simulink model "accumulator"  (R2023b)
settings: Solver=FixedStepAuto  StartTime=0.0  StopTime=10.0  RelTol=1e-3
libraries: c280xlib x26, c2837xDlib x13, canmsglib x8
settings Model: ExtModeTrigDuration=8  Creator=steve  LastModifiedBy=lukeh
settings OptimizationCC: DefaultUnderspecifiedDataType=single  EnhancedBackFolding=on  PassReuseOutputArgsAs=Individual arguments  MaxStackSize=1024  OptimizeBlockOrder=speed  DifferentSizesBufferReuse=on  OptimizationCustomize=off  DenormalBehavior=FlushToZero  EfficientTunableParamExpr=on
settings DebuggingCC: ParameterTunabilityLossMsg=error
settings HardwareCC: ProdBitPerChar=16  ProdBitPerInt=16  ProdBitPerPointer=32  ProdBitPerSizeT=32  ProdBitPerPtrDiffT=32  ProdLargestAtomicInteger=Integer  ProdLargestAtomicFloat=None  ProdWordSize=16  ProdLongLongMode=on  ProdHWDeviceType=Texas Instruments->C2000
settings SFSimCC: MATLABDynamicMemAlloc=off
settings RTWCC: Description=Embedded Coder  SystemTargetFile=ert.tlc  HardwareBoard=TI Delfino F28379D LaunchPad  TemplateMakefile=ert_default_tmf  Toolchain=Texas Instruments Code Composer Studio (C2000)
settings CodeAppCC: ForceParamTrailComments=on  IgnoreCustomStorageClasses=off  OperatorAnnotations=on  SimulinkDataObjDesc=on  SFDataObjDesc=on  InsertBlockDesc=on
settings ERTTargetCC: CodeReplacementLibrary=TI C28x  ExtModeTransport=4  ExtModeStaticAlloc=on  ExtModeAutomaticAllocSize=off  ExtModeMexFile=ext_xcp  ExtModeIntrfLevel=Level2 - Open

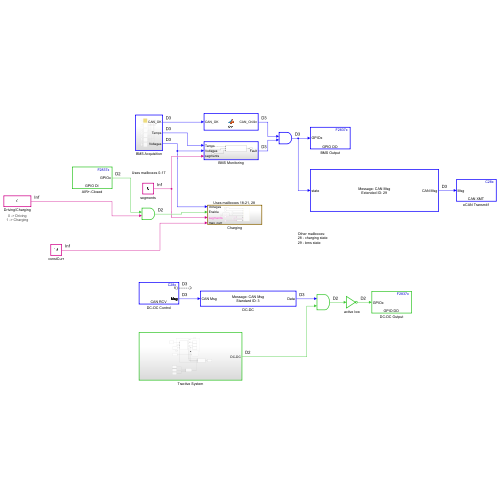
[thumbnail: Simulink's stored preview of the top-level diagram]
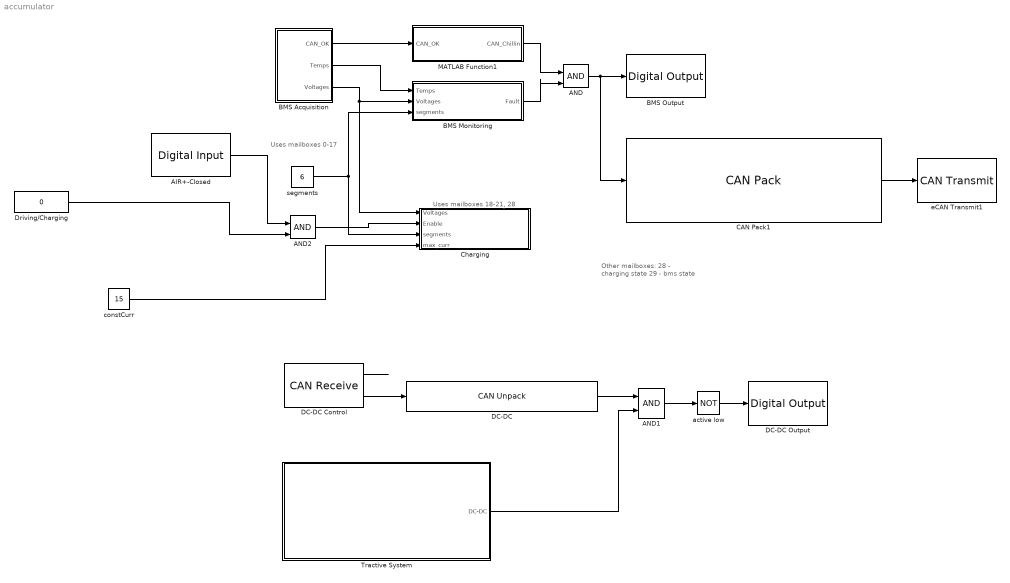
== system accumulator ==
  note: Other mailboxes:
      | 28 - charging state
      | 29 - bms state
  note: Uses mailboxes 18-21, 28
  note: Uses mailboxes 0-17
  AIR+-Closed : c2837xDlib/Digital Input  GPIO_Number=GPIO0~GPIO7  GPIO_Bit0=off  GPIO_Bit1=off  GPIO_Bit2=off  GPIO_Bit3=off  GPIO_Bit4=off  GPIO_Bit5=off  GPIO_Bit6=on  GPIO_Bit7=off  sampleTime=0.1  dataType=auto  GPIO_Bit0_Qualification=Sync to SYSCLKOUT  GPIO_Bit1_Qualification=Sync to SYSCLKOUT  GPIO_Bit2_Qualification=Sync to SYSCLKOUT  GPIO_Bit3_Qualification=Sync to SYSCLKOUT  GPIO_Bit4_Qualification=Sync to SYSCLKOUT  GPIO_Bit5_Qualification=Sync to SYSCLKOUT  GPIO_Bit6_Qualification=Sync to SYSCLKOUT  GPIO_Bit7_Qualification=Sync to SYSCLKOUT  Qualification_Period=-1
  AND : Logic  IconShape=distinctive  AllPortsSameDT=off  OutDataTypeStr=boolean
  AND1 : Logic  IconShape=distinctive  AllPortsSameDT=off  OutDataTypeStr=boolean
  AND2 : Logic  IconShape=distinctive  AllPortsSameDT=off  OutDataTypeStr=boolean
  BMS Acquisition : Subsystem
  BMS Monitoring : Subsystem
  BMS Output : c2837xDlib/Digital Output  GPIO_Number=GPIO56~GPIO63  GPIO_Bit0=off  GPIO_BIT0_Toggle=off  GPIO_Bit1=off  GPIO_BIT1_Toggle=off  GPIO_Bit2=off  GPIO_BIT2_Toggle=off  GPIO_Bit3=off  GPIO_BIT3_Toggle=off  GPIO_Bit4=off  GPIO_BIT4_Toggle=off  GPIO_Bit5=on  GPIO_BIT5_Toggle=off  GPIO_Bit6=off  GPIO_BIT6_Toggle=off  GPIO_Bit7=off  GPIO_BIT7_Toggle=off
  CAN Pack1 : canmsglib/CAN Pack  MsgList=(none)  MsgName=CAN Msg  MsgIDType=Extended (29-bit identifier)  MsgIdentifier=29  MsgLength=8  Remote=off  ApplyMinMax=off  BusOutput=off  SignalInfo={ 'state', '0', '8', 'LE', 'unsigned', 'Standard', '0', '1', '0', '-Inf', 'Inf' }
      settings: DataFormat=manually specified signals
  Charging : Subsystem
  DC-DC : canmsglib/CAN Unpack  MsgList=(none)  MsgName=CAN Msg  MsgIDType=Standard (11-bit identifier)  MsgIdentifier=3  MsgLength=1  SignalInfo={ 'TS_State', '0', '8', 'LE', 'signed', 'Standard', '0', '1', '0', '-Inf', 'Inf' }  IDPort=off  TimestampPort=off  ErrorPort=off  RemotePort=off  LengthPort=off  StatusPort=off  ApplyMinMax=off
      settings: DataFormat=raw data
  DC-DC Control : c280xlib/CAN Receive  chipFamily=C280x  useModule=CAN_B  mailboxNo=30  messageID=3  messageType=Standard (11-bit identifier)  enableAcceptanceFiltering=off  messageIDMask=0  sampleTime=1  dataType=CAN_MESSAGE_TYPE  outputAction=Output last received values  initValue=0  outputMessageID=off  outputMessageLength=off  outputMessageTimeStamp=off  postInterrupt=off  interruptLine=0
  DC-DC Output : c2837xDlib/Digital Output  GPIO_Number=GPIO56~GPIO63  GPIO_Bit0=off  GPIO_BIT0_Toggle=off  GPIO_Bit1=off  GPIO_BIT1_Toggle=off  GPIO_Bit2=on  GPIO_BIT2_Toggle=off  GPIO_Bit3=off  GPIO_BIT3_Toggle=off  GPIO_Bit4=off  GPIO_BIT4_Toggle=off  GPIO_Bit5=off  GPIO_BIT5_Toggle=off  GPIO_Bit6=off  GPIO_BIT6_Toggle=off  GPIO_Bit7=off  GPIO_BIT7_Toggle=off
  Driving/Charging : Constant  Value=0
      settings: AttributesFormatString=|
      | 0 -> Driving
      | 1 -> Charging
  MATLAB Function1 : MATLAB Function  TreatAsAtomicUnit=on
  Tractive System : Subsystem
  active low : Logic  Operator=NOT  IconShape=distinctive  AllPortsSameDT=off  OutDataTypeStr=boolean
  constCurr : Constant  Value=15
  eCAN Transmit1 : c280xlib/CAN Transmit  chipFamily=C280x  useModule=CAN_B  mailboxNo=29  messageID=29  messageType=Extended (29-bit identifier)  enableBlockingMode=off  postInterrupt=off  interruptLine=0
  segments : Constant  Value=6
  wires:
  BMS Acquisition/3(Voltages) -> Charging/1(Voltages), BMS Monitoring/2(Voltages)
  BMS Acquisition/2(Temps) -> BMS Monitoring/1(Temps)
  BMS Acquisition/1(" CAN_OK") -> MATLAB Function1/1(CAN_OK)
  AND/1 -> CAN Pack1/1, BMS Output/1
  MATLAB Function1/1(CAN_Chillin) -> AND/1
  BMS Monitoring/1(Fault) -> AND/2
  CAN Pack1/1 -> eCAN Transmit1/1
  segments/1 -> BMS Monitoring/3(segments), Charging/3(segments)
  DC-DC/1 -> AND1/1
  DC-DC Control/2 -> DC-DC/1
  DC-DC Control/1 -> ?
  AND1/1 -> active low/1
  Tractive System/1(DC-DC) -> AND1/2
  active low/1 -> DC-DC Output/1
  AIR+-Closed/1 -> AND2/1
  AND2/1 -> Charging/2(Enable)
  Driving/Charging/1 -> AND2/2
  constCurr/1 -> Charging/4(max_curr)

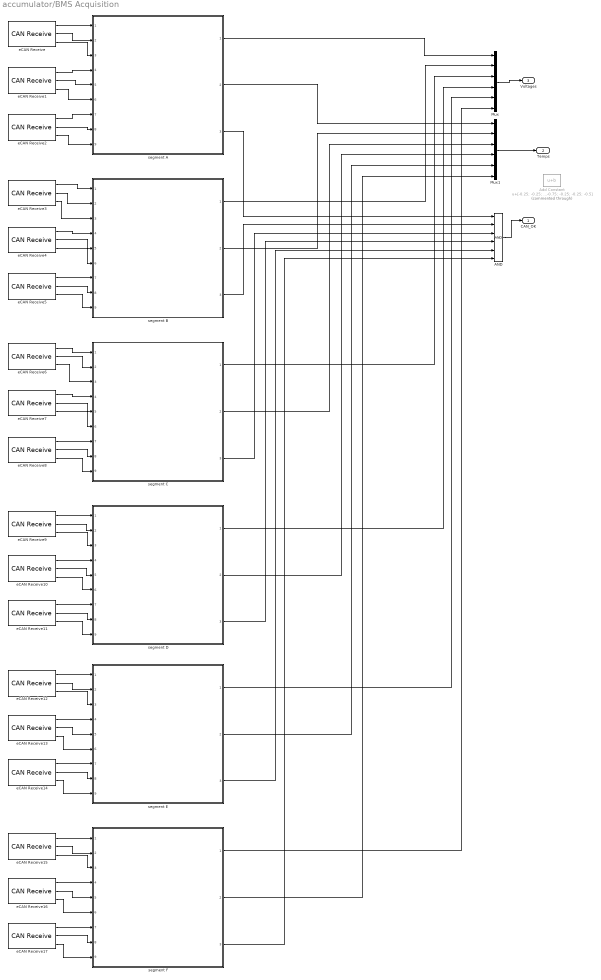
== system accumulator/BMS Acquisition ==
  AND : Logic  Inputs=6  IconShape=distinctive  AllPortsSameDT=off  OutDataTypeStr=boolean
  Add Constant : Bias  Commented=through  Bias=[-0.25; -0.25; -0.25; -1; -0.5; -0.25; -0.5; -0.25; -0.75; -0.5; -0.5; 0; 2.25; 2.25; 2.25; 2.25; 2.25; 2.5; 2.25; 2.5; -1.25; 2.5; 2.25; 2.25; 0.5; 0.5; 0.75; 0.5; 0.75; 1.25; 0.75; 0.5; -1.25; 0.75; 0.75; 0.75; 1.75; 2.5; 2.75; 2.25; 2.5; 2.5; 2.25; 1.75; -2.5; 0; 2.5; 2.75; 1.5; 1.25; 1.25; 0.75; 1.25; 1.25; 1.25; 1.5; -0.75; 1.25; 1.25; 1.25; -0.25; 0; 0; 0; -0.25; -0.5; -0.5; -0.25; -0.75; -0.25; -0.25; -0.5]  SaturateOnIntegerOverflow=off
  Mux : Mux  Inputs=6
  Mux1 : Mux  Inputs=6
  eCAN Receive : c280xlib/CAN Receive  chipFamily=C280x  useModule=CAN_B  mailboxNo=0  messageID=200  messageType=Standard (11-bit identifier)  enableAcceptanceFiltering=off  messageIDMask=0  sampleTime=1  dataType=CAN_MESSAGE_TYPE  outputAction=Reset all fields to zero  initValue=0  outputMessageID=off  outputMessageLength=on  outputMessageTimeStamp=off  postInterrupt=off  interruptLine=0
      settings: AttributesFormatString=ID: %<messageID>, MB: %<mailboxNo>
  eCAN Receive1 : c280xlib/CAN Receive  chipFamily=C280x  useModule=CAN_B  mailboxNo=1  messageID=201  messageType=Standard (11-bit identifier)  enableAcceptanceFiltering=off  messageIDMask=0  sampleTime=1  dataType=CAN_MESSAGE_TYPE  outputAction=Reset all fields to zero  initValue=0  outputMessageID=off  outputMessageLength=on  outputMessageTimeStamp=off  postInterrupt=off  interruptLine=0
      settings: AttributesFormatString=ID: %<messageID>, MB: %<mailboxNo>
  eCAN Receive10 : c280xlib/CAN Receive  chipFamily=C280x  useModule=CAN_B  mailboxNo=10  messageID=210  messageType=Standard (11-bit identifier)  enableAcceptanceFiltering=off  messageIDMask=0  sampleTime=1  dataType=CAN_MESSAGE_TYPE  outputAction=Reset all fields to zero  initValue=0  outputMessageID=off  outputMessageLength=on  outputMessageTimeStamp=off  postInterrupt=off  interruptLine=0
      settings: AttributesFormatString=ID: %<messageID>, MB: %<mailboxNo>
  eCAN Receive11 : c280xlib/CAN Receive  chipFamily=C280x  useModule=CAN_B  mailboxNo=11  messageID=211  messageType=Standard (11-bit identifier)  enableAcceptanceFiltering=off  messageIDMask=0  sampleTime=1  dataType=CAN_MESSAGE_TYPE  outputAction=Reset all fields to zero  initValue=0  outputMessageID=off  outputMessageLength=on  outputMessageTimeStamp=off  postInterrupt=off  interruptLine=0
      settings: AttributesFormatString=ID: %<messageID>, MB: %<mailboxNo>
  eCAN Receive12 : c280xlib/CAN Receive  chipFamily=C280x  useModule=CAN_B  mailboxNo=12  messageID=212  messageType=Standard (11-bit identifier)  enableAcceptanceFiltering=off  messageIDMask=0  sampleTime=1  dataType=CAN_MESSAGE_TYPE  outputAction=Reset all fields to zero  initValue=0  outputMessageID=off  outputMessageLength=on  outputMessageTimeStamp=off  postInterrupt=off  interruptLine=0
      settings: AttributesFormatString=ID: %<messageID>, MB: %<mailboxNo>
  eCAN Receive13 : c280xlib/CAN Receive  chipFamily=C280x  useModule=CAN_B  mailboxNo=13  messageID=213  messageType=Standard (11-bit identifier)  enableAcceptanceFiltering=off  messageIDMask=0  sampleTime=1  dataType=CAN_MESSAGE_TYPE  outputAction=Reset all fields to zero  initValue=0  outputMessageID=off  outputMessageLength=on  outputMessageTimeStamp=off  postInterrupt=off  interruptLine=0
      settings: AttributesFormatString=ID: %<messageID>, MB: %<mailboxNo>
  eCAN Receive14 : c280xlib/CAN Receive  chipFamily=C280x  useModule=CAN_B  mailboxNo=14  messageID=214  messageType=Standard (11-bit identifier)  enableAcceptanceFiltering=off  messageIDMask=0  sampleTime=1  dataType=CAN_MESSAGE_TYPE  outputAction=Reset all fields to zero  initValue=0  outputMessageID=off  outputMessageLength=on  outputMessageTimeStamp=off  postInterrupt=off  interruptLine=0
      settings: AttributesFormatString=ID: %<messageID>, MB: %<mailboxNo>
  eCAN Receive15 : c280xlib/CAN Receive  chipFamily=C280x  useModule=CAN_B  mailboxNo=15  messageID=215  messageType=Standard (11-bit identifier)  enableAcceptanceFiltering=off  messageIDMask=0  sampleTime=1  dataType=CAN_MESSAGE_TYPE  outputAction=Reset all fields to zero  initValue=0  outputMessageID=off  outputMessageLength=on  outputMessageTimeStamp=off  postInterrupt=off  interruptLine=0
      settings: AttributesFormatString=ID: %<messageID>, MB: %<mailboxNo>
  eCAN Receive16 : c280xlib/CAN Receive  chipFamily=C280x  useModule=CAN_B  mailboxNo=16  messageID=216  messageType=Standard (11-bit identifier)  enableAcceptanceFiltering=off  messageIDMask=0  sampleTime=1  dataType=CAN_MESSAGE_TYPE  outputAction=Reset all fields to zero  initValue=0  outputMessageID=off  outputMessageLength=on  outputMessageTimeStamp=off  postInterrupt=off  interruptLine=0
      settings: AttributesFormatString=ID: %<messageID>, MB: %<mailboxNo>
  eCAN Receive17 : c280xlib/CAN Receive  chipFamily=C280x  useModule=CAN_B  mailboxNo=17  messageID=217  messageType=Standard (11-bit identifier)  enableAcceptanceFiltering=off  messageIDMask=0  sampleTime=1  dataType=CAN_MESSAGE_TYPE  outputAction=Reset all fields to zero  initValue=0  outputMessageID=off  outputMessageLength=on  outputMessageTimeStamp=off  postInterrupt=off  interruptLine=0
      settings: AttributesFormatString=ID: %<messageID>, MB: %<mailboxNo>
  eCAN Receive2 : c280xlib/CAN Receive  chipFamily=C280x  useModule=CAN_B  mailboxNo=2  messageID=202  messageType=Standard (11-bit identifier)  enableAcceptanceFiltering=off  messageIDMask=0  sampleTime=1  dataType=CAN_MESSAGE_TYPE  outputAction=Reset all fields to zero  initValue=0  outputMessageID=off  outputMessageLength=on  outputMessageTimeStamp=off  postInterrupt=off  interruptLine=0
      settings: AttributesFormatString=ID: %<messageID>, MB: %<mailboxNo>
  eCAN Receive3 : c280xlib/CAN Receive  chipFamily=C280x  useModule=CAN_B  mailboxNo=3  messageID=203  messageType=Standard (11-bit identifier)  enableAcceptanceFiltering=off  messageIDMask=0  sampleTime=1  dataType=CAN_MESSAGE_TYPE  outputAction=Reset all fields to zero  initValue=0  outputMessageID=off  outputMessageLength=on  outputMessageTimeStamp=off  postInterrupt=off  interruptLine=0
      settings: AttributesFormatString=ID: %<messageID>, MB: %<mailboxNo>
  eCAN Receive4 : c280xlib/CAN Receive  chipFamily=C280x  useModule=CAN_B  mailboxNo=4  messageID=204  messageType=Standard (11-bit identifier)  enableAcceptanceFiltering=off  messageIDMask=0  sampleTime=1  dataType=CAN_MESSAGE_TYPE  outputAction=Reset all fields to zero  initValue=0  outputMessageID=off  outputMessageLength=on  outputMessageTimeStamp=off  postInterrupt=off  interruptLine=0
      settings: AttributesFormatString=ID: %<messageID>, MB: %<mailboxNo>
  eCAN Receive5 : c280xlib/CAN Receive  chipFamily=C280x  useModule=CAN_B  mailboxNo=5  messageID=205  messageType=Standard (11-bit identifier)  enableAcceptanceFiltering=off  messageIDMask=0  sampleTime=1  dataType=CAN_MESSAGE_TYPE  outputAction=Reset all fields to zero  initValue=0  outputMessageID=off  outputMessageLength=on  outputMessageTimeStamp=off  postInterrupt=off  interruptLine=0
      settings: AttributesFormatString=ID: %<messageID>, MB: %<mailboxNo>
  eCAN Receive6 : c280xlib/CAN Receive  chipFamily=C280x  useModule=CAN_B  mailboxNo=6  messageID=206  messageType=Standard (11-bit identifier)  enableAcceptanceFiltering=off  messageIDMask=0  sampleTime=1  dataType=CAN_MESSAGE_TYPE  outputAction=Reset all fields to zero  initValue=0  outputMessageID=off  outputMessageLength=on  outputMessageTimeStamp=off  postInterrupt=off  interruptLine=0
      settings: AttributesFormatString=ID: %<messageID>, MB: %<mailboxNo>
  eCAN Receive7 : c280xlib/CAN Receive  chipFamily=C280x  useModule=CAN_B  mailboxNo=7  messageID=207  messageType=Standard (11-bit identifier)  enableAcceptanceFiltering=off  messageIDMask=0  sampleTime=1  dataType=CAN_MESSAGE_TYPE  outputAction=Reset all fields to zero  initValue=0  outputMessageID=off  outputMessageLength=on  outputMessageTimeStamp=off  postInterrupt=off  interruptLine=0
      settings: AttributesFormatString=ID: %<messageID>, MB: %<mailboxNo>
  eCAN Receive8 : c280xlib/CAN Receive  chipFamily=C280x  useModule=CAN_B  mailboxNo=8  messageID=208  messageType=Standard (11-bit identifier)  enableAcceptanceFiltering=off  messageIDMask=0  sampleTime=1  dataType=CAN_MESSAGE_TYPE  outputAction=Reset all fields to zero  initValue=0  outputMessageID=off  outputMessageLength=on  outputMessageTimeStamp=off  postInterrupt=off  interruptLine=0
      settings: AttributesFormatString=ID: %<messageID>, MB: %<mailboxNo>
  eCAN Receive9 : c280xlib/CAN Receive  chipFamily=C280x  useModule=CAN_B  mailboxNo=9  messageID=209  messageType=Standard (11-bit identifier)  enableAcceptanceFiltering=off  messageIDMask=0  sampleTime=1  dataType=CAN_MESSAGE_TYPE  outputAction=Reset all fields to zero  initValue=0  outputMessageID=off  outputMessageLength=on  outputMessageTimeStamp=off  postInterrupt=off  interruptLine=0
      settings: AttributesFormatString=ID: %<messageID>, MB: %<mailboxNo>
  segment A : Subsystem  ReferencedSubsystem=bms_segment
  segment B : Subsystem  ReferencedSubsystem=bms_segment
  segment C : Subsystem  ReferencedSubsystem=bms_segment
  segment D : Subsystem  ReferencedSubsystem=bms_segment
  segment E : Subsystem  ReferencedSubsystem=bms_segment
  segment F : Subsystem  ReferencedSubsystem=bms_segment
  " CAN_OK" : Outport
  Temps : Outport  Port=2
  Voltages : Outport  Port=3
  wires:
  Mux/1 -> Voltages/1
  eCAN Receive/2 -> segment A/2
  eCAN Receive1/2 -> segment A/5
  eCAN Receive2/2 -> segment A/8
  eCAN Receive/1 -> segment A/1
  eCAN Receive1/1 -> segment A/4
  eCAN Receive2/1 -> segment A/7
  eCAN Receive/3 -> segment A/3
  eCAN Receive1/3 -> segment A/6
  eCAN Receive2/3 -> segment A/9
  AND/1 -> " CAN_OK"/1
  eCAN Receive3/1 -> segment B/1
  eCAN Receive3/2 -> segment B/2
  eCAN Receive4/1 -> segment B/4
  eCAN Receive3/3 -> segment B/3
  eCAN Receive4/2 -> segment B/5
  eCAN Receive4/3 -> segment B/6
  eCAN Receive5/1 -> segment B/7
  eCAN Receive5/2 -> segment B/8
  eCAN Receive5/3 -> segment B/9
  eCAN Receive6/1 -> segment C/1
  eCAN Receive6/2 -> segment C/2
  eCAN Receive6/3 -> segment C/3
  eCAN Receive7/1 -> segment C/4
  eCAN Receive7/2 -> segment C/5
  eCAN Receive7/3 -> segment C/6
  eCAN Receive8/1 -> segment C/7
  eCAN Receive8/2 -> segment C/8
  eCAN Receive8/3 -> segment C/9
  segment A/1 -> Mux/1
  segment A/2 -> Mux1/1
  segment B/1 -> Mux/2
  segment C/1 -> Mux/3
  segment B/2 -> Mux1/2
  segment C/2 -> Mux1/3
  segment A/3 -> AND/1
  segment B/3 -> AND/2
  segment C/3 -> AND/3
  eCAN Receive9/1 -> segment D/1
  eCAN Receive9/2 -> segment D/2
  eCAN Receive9/3 -> segment D/3
  eCAN Receive10/1 -> segment D/4
  eCAN Receive10/2 -> segment D/5
  eCAN Receive10/3 -> segment D/6
  eCAN Receive11/1 -> segment D/7
  eCAN Receive11/2 -> segment D/8
  eCAN Receive11/3 -> segment D/9
  eCAN Receive12/1 -> segment E/1
  eCAN Receive12/2 -> segment E/2
  eCAN Receive12/3 -> segment E/3
  eCAN Receive13/1 -> segment E/4
  eCAN Receive13/2 -> segment E/5
  eCAN Receive13/3 -> segment E/6
  eCAN Receive14/1 -> segment E/7
  eCAN Receive14/2 -> segment E/8
  eCAN Receive14/3 -> segment E/9
  eCAN Receive15/1 -> segment F/1
  eCAN Receive15/2 -> segment F/2
  eCAN Receive15/3 -> segment F/3
  eCAN Receive16/1 -> segment F/4
  eCAN Receive16/2 -> segment F/5
  eCAN Receive16/3 -> segment F/6
  eCAN Receive17/1 -> segment F/7
  eCAN Receive17/2 -> segment F/8
  eCAN Receive17/3 -> segment F/9
  segment D/1 -> Mux/4
  segment E/1 -> Mux/5
  segment F/1 -> Mux/6
  segment D/2 -> Mux1/4
  segment E/2 -> Mux1/5
  segment F/2 -> Mux1/6
  segment D/3 -> AND/4
  segment E/3 -> AND/5
  segment F/3 -> AND/6
  Mux1/1 -> Temps/1

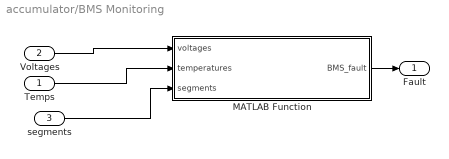
== system accumulator/BMS Monitoring ==
  Temps : Inport
  Voltages : Inport  Port=2
  segments : Inport  Port=3
  MATLAB Function : MATLAB Function  TreatAsAtomicUnit=on
  Fault : Outport
  wires:
  MATLAB Function/1(BMS_fault) -> Fault/1
  Temps/1 -> MATLAB Function/2(temperatures)
  Voltages/1 -> MATLAB Function/1(voltages)
  segments/1 -> MATLAB Function/3(segments)

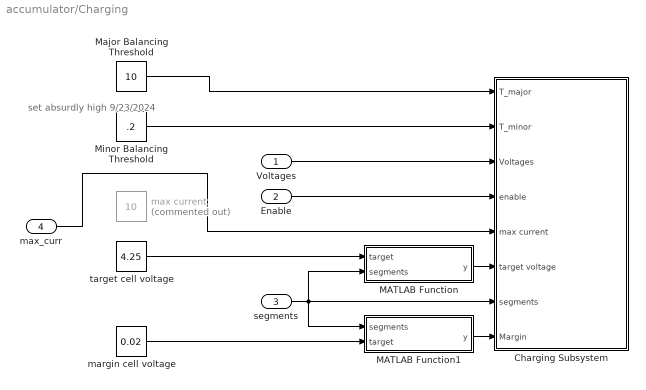
== system accumulator/Charging ==
  note: set absurdly high
      | 9/23/2024
  Voltages : Inport
  Enable : Inport  Port=2
  segments : Inport  Port=3
  max_curr : Inport  Port=4
  Charging Subsystem : Subsystem
  MATLAB Function : MATLAB Function  TreatAsAtomicUnit=on
  MATLAB Function1 : MATLAB Function  TreatAsAtomicUnit=on
  Major Balancing Threshold : Constant  Value=10
  Minor Balancing Threshold : Constant  Value=.2
  margin cell voltage : Constant  Value=0.02
  max current : Constant  Commented=on  Value=10
  target cell voltage : Constant  Value=4.25
  wires:
  Voltages/1 -> Charging Subsystem/3(Voltages)
  Enable/1 -> Charging Subsystem/4(enable)
  max_curr/1 -> Charging Subsystem/5(max current)
  Major Balancing Threshold/1 -> Charging Subsystem/1(T_major)
  Minor Balancing Threshold/1 -> Charging Subsystem/2(T_minor)
  segments/1 -> MATLAB Function/2(segments), MATLAB Function1/1(segments), Charging Subsystem/7(segments)
  target cell voltage/1 -> MATLAB Function/1(target)
  MATLAB Function/1(y) -> Charging Subsystem/6(target voltage)
  MATLAB Function1/1(y) -> Charging Subsystem/8(Margin)
  margin cell voltage/1 -> MATLAB Function1/2(target)

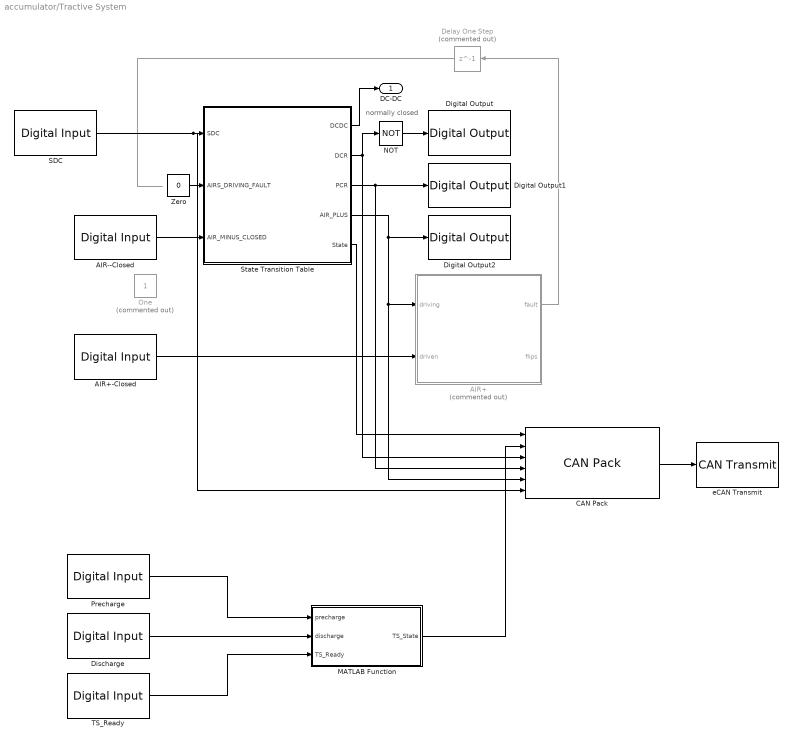
== system accumulator/Tractive System ==
  note: normally closed
  AIR+ : Stateflow chart  Commented=on  TreatAsAtomicUnit=on
      settings: PortSchema="{\"entries\":[{\"content\":{\"sides\":[{\"content\":{\"connectorIds\":[\"In2\",\"In1\"]},\"type\":\"ConnectorPlacement.EquallySpacedRectSide\",\"uuid\":\"9dd53fd1-3ecf-4257-a5bf-55d9d7025cab\"},{\"content\":{\"connectorIds\":[\"Out1\",\"Out2\"],\"side\":\"RIGHT\"},\"type\":\"ConnectorPlacement.EquallySpacedRectSide\",\"uuid\":\"25af85f6-47e3-4235-93a7-84041689babd\"},{\"content\":{\"side\":\"TOP\"},\"type\":\"ConnectorPlacement.EquallySpacedRectSide\",\"uuid\":\"fe47d149-33ed-4c88-9cef-d93cfcf8ed1b\"}]},\"type\":\"ConnectorPlacement.EquallySpacedConnector\",\"uuid\":\"e36ef6f7-edf5-4e9b-b0bb-f3a9ff5ce870\"}],\"packageUris\":[\"http://schema.mathworks.com/mf0/Connector/R2020b\"],\"version\":\"1.0\"}"
  AIR+-Closed : c2837xDlib/Digital Input  GPIO_Number=GPIO0~GPIO7  GPIO_Bit0=off  GPIO_Bit1=off  GPIO_Bit2=off  GPIO_Bit3=off  GPIO_Bit4=off  GPIO_Bit5=off  GPIO_Bit6=on  GPIO_Bit7=off  sampleTime=0.1  dataType=auto  GPIO_Bit0_Qualification=Sync to SYSCLKOUT  GPIO_Bit1_Qualification=Sync to SYSCLKOUT  GPIO_Bit2_Qualification=Sync to SYSCLKOUT  GPIO_Bit3_Qualification=Sync to SYSCLKOUT  GPIO_Bit4_Qualification=Sync to SYSCLKOUT  GPIO_Bit5_Qualification=Sync to SYSCLKOUT  GPIO_Bit6_Qualification=Sync to SYSCLKOUT  GPIO_Bit7_Qualification=Sync to SYSCLKOUT  Qualification_Period=-1
  AIR--Closed : c2837xDlib/Digital Input  GPIO_Number=GPIO0~GPIO7  GPIO_Bit0=off  GPIO_Bit1=off  GPIO_Bit2=off  GPIO_Bit3=off  GPIO_Bit4=off  GPIO_Bit5=off  GPIO_Bit6=off  GPIO_Bit7=on  sampleTime=0.1  dataType=auto  GPIO_Bit0_Qualification=Sync to SYSCLKOUT  GPIO_Bit1_Qualification=Sync to SYSCLKOUT  GPIO_Bit2_Qualification=Sync to SYSCLKOUT  GPIO_Bit3_Qualification=Sync to SYSCLKOUT  GPIO_Bit4_Qualification=Sync to SYSCLKOUT  GPIO_Bit5_Qualification=Sync to SYSCLKOUT  GPIO_Bit6_Qualification=Sync to SYSCLKOUT  GPIO_Bit7_Qualification=Sync to SYSCLKOUT  Qualification_Period=-1
  CAN Pack : canmsglib/CAN Pack  MsgList=(none)  MsgName=CAN Msg  MsgIDType=Standard (11-bit identifier)  MsgIdentifier=2  MsgLength=6  Remote=off  ApplyMinMax=off  BusOutput=off  SignalInfo={ 'SW_State', '0', '8', 'LE', 'signed', 'Standard', '0', '1', '0', '-Inf', 'Inf'; 'HW_State', '8', '8', 'LE', 'signed', 'Standard', '0', '1', '0', '-Inf', 'Inf'; 'DCR', '16', '8', 'LE', 'signed', 'Standard', '0', '1', '0', '-Inf', 'Inf'; 'PCR', '24', '8', 'LE', 'signed', 'Standard', '0', '1', '0', '-Inf', 'Inf'; 'AIR_PLUS', '32', '8', 'LE', 'signed', 'Standard', '0', '1', '0', '-Inf', 'Inf'; 'SDC', '40', '8', 'LE', 'signed', 'Standard', '0', '1', '0', '-Inf', 'Inf' }
      settings: DataFormat=manually specified signals
  Delay One Step : Delay  Commented=on  DelayLength=1
  Digital Output : c2837xDlib/Digital Output  GPIO_Number=GPIO64~GPIO71  GPIO_Bit0=off  GPIO_BIT0_Toggle=off  GPIO_Bit1=off  GPIO_BIT1_Toggle=off  GPIO_Bit2=on  GPIO_BIT2_Toggle=off  GPIO_Bit3=off  GPIO_BIT3_Toggle=off  GPIO_Bit4=off  GPIO_BIT4_Toggle=off  GPIO_Bit5=off  GPIO_BIT5_Toggle=off  GPIO_Bit6=off  GPIO_BIT6_Toggle=off  GPIO_Bit7=off  GPIO_BIT7_Toggle=off
  Digital Output1 : c2837xDlib/Digital Output  GPIO_Number=GPIO128~GPIO135  GPIO_Bit0=off  GPIO_BIT0_Toggle=off  GPIO_Bit1=off  GPIO_BIT1_Toggle=off  GPIO_Bit2=off  GPIO_BIT2_Toggle=off  GPIO_Bit3=on  GPIO_BIT3_Toggle=off  GPIO_Bit4=off  GPIO_BIT4_Toggle=off  GPIO_Bit5=off  GPIO_BIT5_Toggle=off  GPIO_Bit6=off  GPIO_BIT6_Toggle=off  GPIO_Bit7=off  GPIO_BIT7_Toggle=off
  Digital Output2 : c2837xDlib/Digital Output  GPIO_Number=GPIO120~GPIO127  GPIO_Bit0=off  GPIO_BIT0_Toggle=off  GPIO_Bit1=off  GPIO_BIT1_Toggle=off  GPIO_Bit2=off  GPIO_BIT2_Toggle=off  GPIO_Bit3=on  GPIO_BIT3_Toggle=off  GPIO_Bit4=off  GPIO_BIT4_Toggle=off  GPIO_Bit5=off  GPIO_BIT5_Toggle=off  GPIO_Bit6=off  GPIO_BIT6_Toggle=off  GPIO_Bit7=off  GPIO_BIT7_Toggle=off
  Discharge : c2837xDlib/Digital Input  GPIO_Number=GPIO8~GPIO15  GPIO_Bit0=off  GPIO_Bit1=off  GPIO_Bit2=off  GPIO_Bit3=on  GPIO_Bit4=off  GPIO_Bit5=off  GPIO_Bit6=off  GPIO_Bit7=off  sampleTime=0.1  dataType=auto  GPIO_Bit0_Qualification=Sync to SYSCLKOUT  GPIO_Bit1_Qualification=Sync to SYSCLKOUT  GPIO_Bit2_Qualification=Sync to SYSCLKOUT  GPIO_Bit3_Qualification=Sync to SYSCLKOUT  GPIO_Bit4_Qualification=Sync to SYSCLKOUT  GPIO_Bit5_Qualification=Sync to SYSCLKOUT  GPIO_Bit6_Qualification=Sync to SYSCLKOUT  GPIO_Bit7_Qualification=Sync to SYSCLKOUT  Qualification_Period=-1
  MATLAB Function : MATLAB Function  TreatAsAtomicUnit=on
  NOT : Logic  Operator=NOT  IconShape=distinctive  AllPortsSameDT=off  OutDataTypeStr=boolean
  One : Constant  Commented=on  OutDataTypeStr=Inherit: Inherit via back propagation
  Precharge : c2837xDlib/Digital Input  GPIO_Number=GPIO8~GPIO15  GPIO_Bit0=off  GPIO_Bit1=off  GPIO_Bit2=off  GPIO_Bit3=off  GPIO_Bit4=off  GPIO_Bit5=off  GPIO_Bit6=on  GPIO_Bit7=off  sampleTime=0.1  dataType=auto  GPIO_Bit0_Qualification=Sync to SYSCLKOUT  GPIO_Bit1_Qualification=Sync to SYSCLKOUT  GPIO_Bit2_Qualification=Sync to SYSCLKOUT  GPIO_Bit3_Qualification=Sync to SYSCLKOUT  GPIO_Bit4_Qualification=Sync to SYSCLKOUT  GPIO_Bit5_Qualification=Sync to SYSCLKOUT  GPIO_Bit6_Qualification=Sync to SYSCLKOUT  GPIO_Bit7_Qualification=Sync to SYSCLKOUT  Qualification_Period=-1
  SDC : c2837xDlib/Digital Input  GPIO_Number=GPIO24~GPIO31  GPIO_Bit0=on  GPIO_Bit1=off  GPIO_Bit2=off  GPIO_Bit3=off  GPIO_Bit4=off  GPIO_Bit5=off  GPIO_Bit6=off  GPIO_Bit7=off  sampleTime=0.1  dataType=auto  GPIO_Bit0_Qualification=Sync to SYSCLKOUT  GPIO_Bit1_Qualification=Sync to SYSCLKOUT  GPIO_Bit2_Qualification=Sync to SYSCLKOUT  GPIO_Bit3_Qualification=Sync to SYSCLKOUT  GPIO_Bit4_Qualification=Sync to SYSCLKOUT  GPIO_Bit5_Qualification=Sync to SYSCLKOUT  GPIO_Bit6_Qualification=Sync to SYSCLKOUT  GPIO_Bit7_Qualification=Sync to SYSCLKOUT  Qualification_Period=-1
  State Transition Table : State Transition Table  TreatAsAtomicUnit=on
      settings: PortSchema="{\"entries\":[{\"content\":{\"sides\":[{\"content\":{\"connectorIds\":[\"In1\",\"In3\",\"In2\"]},\"type\":\"ConnectorPlacement.EquallySpacedRectSide\",\"uuid\":\"588cd4c7-dba0-48db-9820-dba2fd8491b3\"},{\"content\":{\"connectorIds\":[\"Out1\",\"Out2\",\"Out3\",\"Out4\",\"Out5\"],\"side\":\"RIGHT\"},\"type\":\"ConnectorPlacement.EquallySpacedRectSide\",\"uuid\":\"afcbba97-d13d-4a71-ab90-836a8403ff14\"},{\"content\":{\"side\":\"TOP\"},\"type\":\"ConnectorPlacement.EquallySpacedRectSide\",\"uuid\":\"fcc09a8a-eb74-45bd-9fb8-425b0c125d01\"}]},\"type\":\"ConnectorPlacement.EquallySpacedConnector\",\"uuid\":\"9519508f-2f94-439f-97d1-f6b865d2cc07\"}],\"packageUris\":[\"http://schema.mathworks.com/mf0/Connector/R2020b\"],\"version\":\"1.0\"}"
  TS_Ready : c2837xDlib/Digital Input  GPIO_Number=GPIO8~GPIO15  GPIO_Bit0=off  GPIO_Bit1=off  GPIO_Bit2=on  GPIO_Bit3=off  GPIO_Bit4=off  GPIO_Bit5=off  GPIO_Bit6=off  GPIO_Bit7=off  sampleTime=0.1  dataType=auto  GPIO_Bit0_Qualification=Sync to SYSCLKOUT  GPIO_Bit1_Qualification=Sync to SYSCLKOUT  GPIO_Bit2_Qualification=Sync to SYSCLKOUT  GPIO_Bit3_Qualification=Sync to SYSCLKOUT  GPIO_Bit4_Qualification=Sync to SYSCLKOUT  GPIO_Bit5_Qualification=Sync to SYSCLKOUT  GPIO_Bit6_Qualification=Sync to SYSCLKOUT  GPIO_Bit7_Qualification=Sync to SYSCLKOUT  Qualification_Period=-1
  Zero : Constant  Value=0  OutDataTypeStr=Inherit: Inherit via back propagation
  eCAN Transmit : c280xlib/CAN Transmit  chipFamily=C280x  useModule=CAN_B  mailboxNo=31  messageID=2  messageType=Standard (11-bit identifier)  enableBlockingMode=off  postInterrupt=off  interruptLine=0
  DC-DC : Outport
  wires:
  State Transition Table/4(AIR_PLUS) -> CAN Pack/5, AIR+/2(driving), Digital Output2/1
  AIR+-Closed/1 -> AIR+/1(driven)
  AIR--Closed/1 -> State Transition Table/2(AIR_MINUS_CLOSED)
  AIR+/1(fault) -> Delay One Step/1
  Delay One Step/1 -> ?
  SDC/1 -> CAN Pack/6, State Transition Table/1(SDC)
  State Transition Table/2(DCR) -> NOT/1, CAN Pack/3
  State Transition Table/3(PCR) -> CAN Pack/4, Digital Output1/1
  Zero/1 -> State Transition Table/3(AIRS_DRIVING_FAULT)
  NOT/1 -> Digital Output/1
  State Transition Table/5(State) -> CAN Pack/1
  CAN Pack/1 -> eCAN Transmit/1
  Precharge/1 -> MATLAB Function/1(precharge)
  Discharge/1 -> MATLAB Function/2(discharge)
  TS_Ready/1 -> MATLAB Function/3(TS_Ready)
  MATLAB Function/1(TS_State) -> CAN Pack/2
  State Transition Table/1(DCDC) -> DC-DC/1

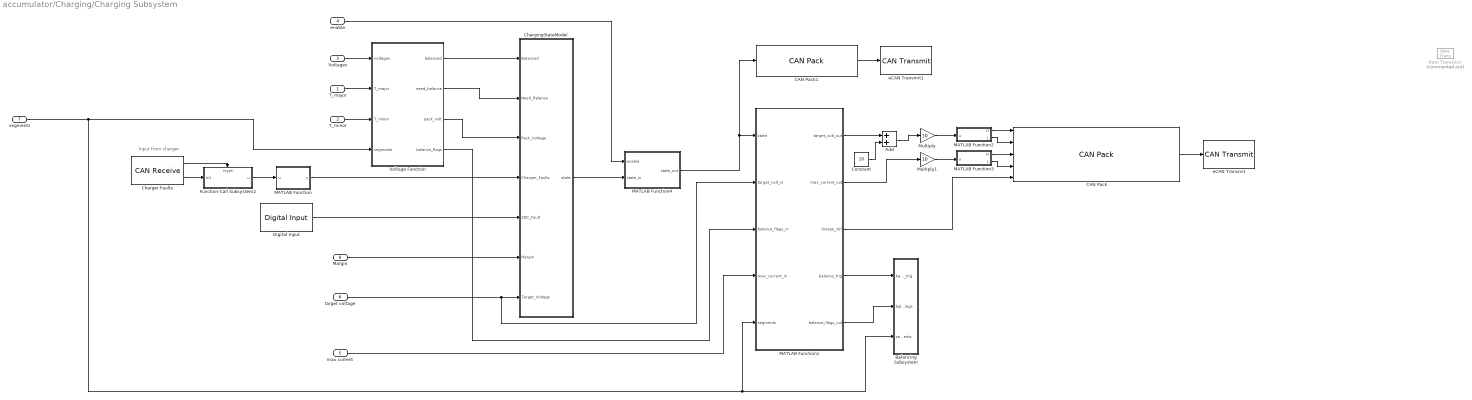
== system accumulator/Charging/Charging Subsystem ==
  note: Input from charger
  T_major : Inport
  T_minor : Inport  Port=2
  Voltages : Inport  Port=3
  enable : Inport  Port=4
  max current : Inport  Port=5
  target voltage : Inport  Port=6
  segments : Inport  Port=7
  Margin : Inport  Port=8
  Add : Sum
  Balancing Subsystem : Subsystem  TreatAsAtomicUnit=on
  CAN Pack : canmsglib/CAN Pack  MsgList=(none)  MsgName=CAN Msg  MsgIDType=Extended (29-bit identifier)  MsgIdentifier=403105780  MsgLength=8  Remote=off  ApplyMinMax=off  BusOutput=off  SignalInfo={ 'MaxVoltageHigh', '0', '8', 'LE', 'unsigned', 'Standard', '0', '1', '0', '-Inf', 'Inf'; 'MaxVoltageLow', '8', '8', 'LE', 'unsigned', 'Standard', '0', '1', '0', '-Inf', 'Inf'; 'MaxCurrentHigh', '16', '8', 'LE', 'unsigned', 'Standard', '0', '1', '0', '-Inf', 'Inf'; 'MaxCurrentLow', '24', '8', 'LE', 'unsigned', 'Standard', '0', '1', '0', '-Inf', 'Inf'; 'CTRL', '32', '8', 'LE', 'unsigned', 'Standard', '0', '1', '0', '-Inf', 'Inf' }
      settings: DataFormat=manually specified signals
  CAN Pack1 : canmsglib/CAN Pack  MsgList=(none)  MsgName=CAN Msg  MsgIDType=Extended (29-bit identifier)  MsgIdentifier=28  MsgLength=8  Remote=off  ApplyMinMax=off  BusOutput=off  SignalInfo={ 'state', '0', '8', 'LE', 'unsigned', 'Standard', '0', '1', '0', '-Inf', 'Inf' }
      settings: DataFormat=manually specified signals
  Charger Faults : c280xlib/CAN Receive  chipFamily=C280x  useModule=CAN_B  mailboxNo=18  messageID=419385573  messageType=Extended (29-bit identifier)  enableAcceptanceFiltering=off  messageIDMask=0  sampleTime=.01  dataType=CAN_MESSAGE_TYPE  outputAction=Output last received values  initValue=0  outputMessageID=off  outputMessageLength=off  outputMessageTimeStamp=off  postInterrupt=off  interruptLine=0
  ChargingStateModel : Stateflow chart  TreatAsAtomicUnit=on  SystemSampleTime=0.01
      settings: RTWSystemCode=Inline  RTWFcnNameOpts=Use subsystem name  RTWFileNameOpts=Use subsystem name  PortSchema="{\"entries\":[{\"content\":{\"sides\":[{\"content\":{\"connectorIds\":[\"In1\",\"In6\",\"In5\",\"In3\",\"In7\",\"In2\",\"In4\"]},\"type\":\"ConnectorPlacement.EquallySpacedRectSide\",\"uuid\":\"e489c846-491e-4e82-9c5f-b669d7c96954\"},{\"content\":{\"connectorIds\":[\"Out1\"],\"side\":\"RIGHT\"},\"type\":\"ConnectorPlacement.EquallySpacedRectSide\",\"uuid\":\"cbb46da5-6eb6-44f9-baf3-a24ec6c96225\"},{\"content\":{\"connectorIds\":[],\"side\":\"TOP\"},\"type\":\"ConnectorPlacement.EquallySpacedRectSide\",\"uuid\":\"c6202e3b-aafb-4b81-a309-4cc98c9bb853\"},{\"content\":{\"connectorIds\":[],\"side\":\"BOTTOM\"},\"type\":\"ConnectorPlacement.EquallySpacedRectSide\",\"uuid\":\"d6a20d7c-ea9b-4afd-8884-952a45f498ea\"}]},\"type\":\"ConnectorPlacement.EquallySpacedConnector\",\"uuid\":\"7c3bea70-19b9-40c4-b7cb-79b1c3f0d3c0\"}],\"packageUris\":[\"http://schema.mathworks.com/mf0/Connector/R2020b\"],\"version\":\"1.0\"}"
  Constant : Constant  Value=10
  Digital Input : c2837xDlib/Digital Input  GPIO_Number=GPIO8~GPIO15  GPIO_Bit0=on  GPIO_Bit1=off  GPIO_Bit2=off  GPIO_Bit3=off  GPIO_Bit4=off  GPIO_Bit5=off  GPIO_Bit6=off  GPIO_Bit7=off  sampleTime=0.1  dataType=auto  GPIO_Bit0_Qualification=Sync to SYSCLKOUT  GPIO_Bit1_Qualification=Sync to SYSCLKOUT  GPIO_Bit2_Qualification=Sync to SYSCLKOUT  GPIO_Bit3_Qualification=Sync to SYSCLKOUT  GPIO_Bit4_Qualification=Sync to SYSCLKOUT  GPIO_Bit5_Qualification=Sync to SYSCLKOUT  GPIO_Bit6_Qualification=Sync to SYSCLKOUT  GPIO_Bit7_Qualification=Sync to SYSCLKOUT  Qualification_Period=-1
  Function-Call Subsystem2 : Subsystem  TreatAsAtomicUnit=on
  MATLAB Function : MATLAB Function  TreatAsAtomicUnit=on
  MATLAB Function1 : MATLAB Function  TreatAsAtomicUnit=on
  MATLAB Function2 : MATLAB Function  TreatAsAtomicUnit=on
  MATLAB Function3 : MATLAB Function  TreatAsAtomicUnit=on
  MATLAB Function4 : MATLAB Function  TreatAsAtomicUnit=on
  Multiply : Gain  Gain=10
  Multiply1 : Gain  Gain=10
  Rate Transition : RateTransition  Commented=on  OutPortSampleTime=.5
  Voltage Function : MATLAB Function  TreatAsAtomicUnit=on
  eCAN Transmit : c280xlib/CAN Transmit  chipFamily=C280x  useModule=CAN_B  mailboxNo=19  messageID=403105780  messageType=Extended (29-bit identifier)  enableBlockingMode=off  postInterrupt=off  interruptLine=0
  eCAN Transmit1 : c280xlib/CAN Transmit  chipFamily=C280x  useModule=CAN_B  mailboxNo=28  messageID=28  messageType=Extended (29-bit identifier)  enableBlockingMode=off  postInterrupt=off  interruptLine=0
  wires:
  ChargingStateModel/1(state) -> MATLAB Function4/2(state_in)
  Voltage Function/3(pack_volt) -> ChargingStateModel/5(Pack_Voltage)
  Voltages/1 -> Voltage Function/1(voltages)
  Charger Faults/2 -> Function-Call Subsystem2/1(In1)
  Charger Faults/1 -> Function-Call Subsystem2/Trigger
  Function-Call Subsystem2/1(u) -> MATLAB Function/1(u)
  MATLAB Function/1(y) -> ChargingStateModel/3(Charger_Faults)
  Digital Input/1 -> ChargingStateModel/7(SDC_Fault)
  MATLAB Function4/1(state_out) -> MATLAB Function1/1(state), CAN Pack1/1
  Multiply/1 -> MATLAB Function2/1(u)
  CAN Pack/1 -> eCAN Transmit/1
  Multiply1/1 -> MATLAB Function3/1(u)
  MATLAB Function2/1(H) -> CAN Pack/1
  MATLAB Function3/1(H) -> CAN Pack/3
  MATLAB Function2/2(L) -> CAN Pack/2
  MATLAB Function3/2(L) -> CAN Pack/4
  max current/1 -> MATLAB Function1/4(max_current_in)
  MATLAB Function1/2(max_current_out) -> Multiply1/1
  MATLAB Function1/3(charge_ctrl) -> CAN Pack/5
  target voltage/1 -> MATLAB Function1/2(target_volt_in), ChargingStateModel/4(Target_Voltage)
  Voltage Function/1(balanced) -> ChargingStateModel/1(Balanced)
  Voltage Function/2(need_balance) -> ChargingStateModel/6(Need_Balance)
  Margin/1 -> ChargingStateModel/2(Margin)
  T_major/1 -> Voltage Function/2(T_major)
  T_minor/1 -> Voltage Function/3(T_minor)
  MATLAB Function1/4(balance_trig) -> Balancing Subsystem/1(balance_trig)
  Voltage Function/4(balance_flags) -> MATLAB Function1/3(balance_flags_in)
  CAN Pack1/1 -> eCAN Transmit1/1
  enable/1 -> MATLAB Function4/1(enable)
  MATLAB Function1/5(balance_flags_out) -> Balancing Subsystem/2(balance_flags)
  segments/1 -> MATLAB Function1/5(segments), Balancing Subsystem/3(segments), Voltage Function/4(segments)
  MATLAB Function1/1(target_volt_out) -> Add/1
  Add/1 -> Multiply/1
  Constant/1 -> Add/2

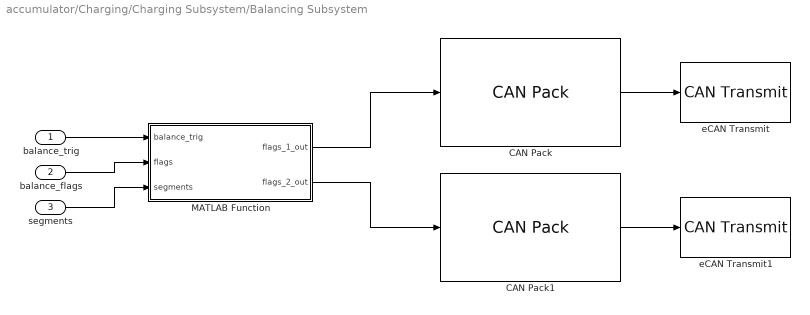
== system accumulator/Charging/Charging Subsystem/Balancing Subsystem ==
  balance_trig : Inport
  balance_flags : Inport  Port=2
  segments : Inport  Port=3
  CAN Pack : canmsglib/CAN Pack  MsgList=(none)  MsgName=CAN Msg  MsgIDType=Standard (11-bit identifier)  MsgIdentifier=220  MsgLength=8  Remote=off  ApplyMinMax=off  BusOutput=off  SignalInfo={}
      settings: LibrarySourceBlock=c2000lib/Target Communication/CAN Pack  DataFormat=raw data
  CAN Pack1 : canmsglib/CAN Pack  MsgList=(none)  MsgName=CAN Msg  MsgIDType=Standard (11-bit identifier)  MsgIdentifier=221  MsgLength=8  Remote=off  ApplyMinMax=off  BusOutput=off  SignalInfo={}
      settings: LibrarySourceBlock=c2000lib/Target Communication/CAN Pack  DataFormat=raw data
  MATLAB Function : MATLAB Function  TreatAsAtomicUnit=on
  eCAN Transmit : c280xlib/CAN Transmit  chipFamily=C280x  useModule=CAN_B  mailboxNo=20  messageID=220  messageType=Standard (11-bit identifier)  enableBlockingMode=off  postInterrupt=off  interruptLine=0
  eCAN Transmit1 : c280xlib/CAN Transmit  chipFamily=C280x  useModule=CAN_B  mailboxNo=21  messageID=221  messageType=Standard (11-bit identifier)  enableBlockingMode=off  postInterrupt=off  interruptLine=0
  wires:
  balance_flags/1 -> MATLAB Function/2(flags)
  MATLAB Function/1(flags_1_out) -> CAN Pack/1
  CAN Pack/1 -> eCAN Transmit/1
  MATLAB Function/2(flags_2_out) -> CAN Pack1/1
  CAN Pack1/1 -> eCAN Transmit1/1
  balance_trig/1 -> MATLAB Function/1(balance_trig)
  segments/1 -> MATLAB Function/3(segments)

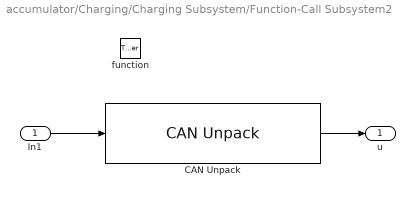
== system accumulator/Charging/Charging Subsystem/Function-Call Subsystem2 ==
  In1 : Inport
  function : TriggerPort  TriggerType=function-call  VariantControl=(inherit)
  CAN Unpack : canmsglib/CAN Unpack  MsgList=(none)  MsgName=CAN Msg  MsgIDType=Extended (29-bit identifier)  MsgIdentifier=419385573  MsgLength=8  SignalInfo={ 'Signal1', '0', '8', 'LE', 'signed', 'Standard', '0', '1', '0', '-Inf', 'Inf' }  IDPort=off  TimestampPort=off  ErrorPort=off  RemotePort=off  LengthPort=off  StatusPort=off  ApplyMinMax=off
      settings: DataFormat=raw data
  u : Outport
  wires:
  In1/1 -> CAN Unpack/1
  CAN Unpack/1 -> u/1

== stateflow chart accumulator/Tractive System/AIR+ ==
  state Low_Fault
    fault = 4;
  state High
    fault = 0;
  state Up_Fault
    fault = 1;
  state Up
    fault = 0;
  state Down
    fault = 0;
  state Down_Fault
    fault = 2;
  state Low
    fault = 0;
  state High_Fault
    fault = 3;
  High -> Low_Fault [order 2] : [~driven]
  High -> Down [order 1] : [~driving && driven]
  Up -> High [order 1] : [driving && driven]
  Up -> Down [order 3] : [~driving]{flips=flips+1}
  Up -> Up_Fault [order 2] : [after(100, msec)]
  Down -> Down_Fault [order 2] : [after(100, msec)]
  Down -> Up [order 3] : [driving]{flips=flips+1}
  (default) -> Low
  Low -> Up [order 1] : [driving && ~driven]
  Down -> Low [order 1] : [~driving && ~driven]
  Low -> High_Fault [order 2] : [driven]
  data: driven input; driving input; fault output; flips output

== stateflow chart accumulator/Tractive System/State Transition Table ==
  state Start_Discharge
    State = 0;
    DCR = 1;
    PCR = 0;
    AIR_PLUS = 0;
    DCDC = 0;
  state Discharge
    State = 1;
    DCR = 0;
    PCR = 0;
    AIR_PLUS = 0;
    DCDC = 0;
    on after(DEAD_MSEC, msec):
    DCR = 1;
  state Precharge
    State = 2;
    DCR = 0;
    PCR = 0;
    AIR_PLUS = 0;
    DCDC = 0;
    on after(DEAD_MSEC, msec):
    PCR = 1;
  state TS_Ready
    State = 3;
    DCR = 0;
    PCR = 1;
    AIR_PLUS = 1;
    DCDC = 1;
  state AK_Discharge
    State = -1;
    DCR = 0;
    PCR = 0;
    AIR_PLUS = 0;
    DCDC = 0;
    on after(DEAD_MSEC, msec):
    DCR = 1;
  (default) -> Start_Discharge
  Start_Discharge -> (junction 65) [order 2] : [SDC && AIR_MINUS_CLOSED]
  (junction 65) -> (junction 63)
  Start_Discharge -> (junction 78) [order 1] : [AIRS_DRIVING_FAULT]
  (junction 78) -> (junction 85)
  (junction 69) -> Discharge
  Discharge -> (junction 85) [order 1] : [AIRS_DRIVING_FAULT]
  (junction 71) -> (junction 69)
  (junction 85) -> (junction 92)
  Discharge -> (junction 92) [order 2] : [ak_counter > AK_THRESHOLD]
  (junction 92) -> (junction 82)
  Discharge -> Precharge [order 3] : [SDC && AIR_MINUS_CLOSED]
  Precharge -> Discharge [order 2] : [~SDC]
      | {ak_counter = ak_counter + 1;}
  (junction 63) -> Precharge
  Precharge -> (junction 82) [order 1] : [AIRS_DRIVING_FAULT]
  (junction 82) -> (junction 76)
  Precharge -> TS_Ready [order 3] : [after(PC_SEC, sec)]
  TS_Ready -> (junction 71) [order 2] : [~SDC]
  TS_Ready -> AK_Discharge [order 1] : [AIRS_DRIVING_FAULT]
  (junction 76) -> AK_Discharge
  data: DCDC output; DCR output; PCR output; AIR_PLUS output; SDC input; AIR_MINUS_CLOSED input; PC_SEC constant double =9.24; DEAD_MSEC constant double =500; AIRS_DRIVING_FAULT input; ak_counter local =0; AK_THRESHOLD constant double =4; State output

== matlab function accumulator/BMS Monitoring/MATLAB Function ==
  data: voltages input; BMS_fault output; temperatures input; segments input
% checks if there are out of range temperatures or voltages for a segment's
% worth of battery modules
function BMS_fault = BMSfault(voltages, temperatures, segments)

% countVoltErrs will retain its value across multiple function calls
persistent countVoltErrs countTempErrs
if isempty(countVoltErrs)
    countVoltErrs = zeros(72,1);
    countTempErrs = zeros(72,1);
end

BMS_fault=true; % 1 means not faulted

voltErrThresh = 3; % the number of voltage faulse readings before an error is sent,
totalVoltErr = 0;
totalVoltErrThresh = 3; % the number of bad sensors accepted at once without fault

% checks if there are multiple voltage errrors in a row
for i = 1:(segments*12)
    if(voltages(i)>4.25||voltages(i)<2.5) 
        % voltage value transmitted on the CAN message is the actual voltages of the cells
        countVoltErrs(i) = countVoltErrs(i) + 1; % if there is an error, inc counter
    else 
        countVoltErrs(i) = 0; % if no errors, reset the given counter
    end
    if(countVoltErrs(i) > voltErrThresh) % if exceeding threshold, trigger error
        totalVoltErr = totalVoltErr + 1;
        if(totalVoltErr > totalVoltErrThresh)
            BMS_fault=false;
        end
    end
end

tempErrThresh = 3; % the number of false readings issues before an error is sent, was 3 but changed to 6 rosnel
totalTempErr = 0;
totalTempErrThresh = 12*segments*0.1;

for i = 1:(segments*12)
    if(temperatures(i)>=60) % T is in Celcius. changed to 60C by rosnel, may 31 
        countTempErrs(i) = countTempErrs(i) + 1; % if there is an error, inc counter
    else 
        countTempErrs(i) = 0; % if no errors, reset the given counter
    end
    if(countTempErrs(i) > tempErrThresh) % if exceeding threshold, trigger error
        totalTempErr = totalTempErr + 1;
        if(totalTempErr > totalTempErrThresh)
            BMS_fault=false;
        end
    end
end

end

== matlab function accumulator/Tractive System/MATLAB Function ==
  data: precharge input; discharge input; TS_Ready input; TS_State output
function TS_State = fcn(precharge, discharge, TS_Ready)
%#codegen
a = precharge + discharge + TS_Ready;
if ((precharge && discharge) || (discharge && TS_Ready))
    TS_State = 0;
else
    if(precharge && TS_Ready)
        TS_State=2;
    elseif(discharge==1)
        TS_State=1;
    else
        TS_State=3;
    end
end

== stateflow chart accumulator/Charging/Charging Subsystem/ChargingStateModel ==
  state Cool_Down
    state=7;
  state Change_State
    state=8;
  state Balance_Module
    state=2;
  state Wait
    state=5;
  state Charge_Complete
    state=6;
  state Start
    state=0;
  state Charging
    state=1;
  state SDC_Fault
    state=3;
  state Charger_Fault
    state=4;
  Charging -> Cool_Down [order 3] : after(600,sec)
  Balance_Module -> Cool_Down [order 2] : after(120,sec)
  Cool_Down -> Change_State : after(5,sec)
  Change_State -> Wait [order 3] : [Pack_Voltage >= Target_Voltage]
  Change_State -> Charging [order 2] : [Balanced == 1 && Pack_Voltage < Target_Voltage]
  Change_State -> Balance_Module [order 1] : [Need_Balance == 1]
  Wait -> Balance_Module [order 1] : [Balanced==0]
  Wait -> Charge_Complete [order 3] : after(60, sec)
  (default) -> Start
  Balance_Module -> SDC_Fault [order 1] : [SDC_Fault == 1]
  Balance_Module -> Charger_Fault [order 3] : [Charger_Faults(1)==1]
  Start -> Charging : [SDC_Fault == 0]
  Wait -> Charging [order 5] : [Pack_Voltage < Target_Voltage - Margin]
  Wait -> SDC_Fault [order 2] : [SDC_Fault == 1]
  Wait -> Charger_Fault [order 4] : [Charger_Faults(1)==1]
  Charging -> Charger_Fault [order 2] : [Charger_Faults(1)==1]
  Charging -> SDC_Fault [order 1] : [SDC_Fault == 1]
  data: Balanced input; Margin input; Charger_Faults input; Target_Voltage input; Pack_Voltage input; Need_Balance input; SDC_Fault input; state output

== matlab function accumulator/Charging/Charging Subsystem/Voltage Function ==
  data: balanced output; need_balance output; voltages input; pack_volt output; T_major input; T_minor input; balance_flags output; segments input

function [balanced, need_balance, pack_volt, balance_flags]  = volt_fun(voltages, T_major, T_minor, segments)

balanced = 1; % 1 means balanced, all of the voltages are within Tminor from min voltage
need_balance = 0; % need_balance=1 means any of the voltages is at least Tmajor above min voltage

minVoltage = min(voltages);
balance_flags = zeros(72, 1);

for i = 1:(segments*12)
    if(voltages(i) - minVoltage > T_major) 
        need_balance = 1;
    end
    if(voltages(i) - minVoltage > T_minor)
        balanced = 0;
        balance_flags(i) = 1;
    end
end

% now calculate the voltage of the entire pack
% simply sum all individual voltages

pack_volt = sum(voltages);
% the summed voltage should be comparable to target voltage

== matlab function accumulator/Charging/Charging Subsystem/MATLAB Function4 ==
  data: enable input; state_out output; state_in input
function state_out = fcn(enable, state_in)
    if enable == 0
        state_out = 6;
    else
        state_out = state_in;
    end

== matlab function accumulator/MATLAB Function1 ==
  data: CAN_OK input; CAN_Chillin output
function CAN_Chillin = fcn(CAN_OK)

persistent countCANTimeout %CAN_SAD
if isempty(countCANTimeout) %initialize persistant variable
    countCANTimeout = 0;
end

CAN_Chillin = true; % 1 means not faulted

CANThresh = 2; % the number of CAN problems before an error is sent

% checks if there are multiple CAN timeout errrors in a row
if(CAN_OK == 0) 
    countCANTimeout = countCANTimeout + 1; % if there is an error, inc counter
else 
    countCANTimeout = 0; % if no errors, reset the counter
end

if(countCANTimeout > CANThresh) % if exceeding threshold, trigger error
    CAN_Chillin=false;
end

end

== matlab function accumulator/Charging/Charging Subsystem/MATLAB Function ==
  data: u input; y output
function y = fcn(u)
    if u(5)>0
        y = 1;
    else
        y = 0;
    end
end

== matlab function accumulator/Charging/MATLAB Function ==
  data: target input; y output; segments input
function y = fcn(target, segments)
    y = 12*segments*target;

== matlab function accumulator/Charging/MATLAB Function1 ==
  data: segments input; target input; y output
function y = fcn(segments, target)
    y = 12*segments*target;

== matlab function accumulator/Charging/Charging Subsystem/MATLAB Function1 ==
  data: state input; target_volt_in input; balance_flags_in input; target_volt_out output; max_current_in input; max_current_out output; charge_ctrl output; balance_trig output; balance_flags_out output size=72; segments input
function [target_volt_out, max_current_out, charge_ctrl, balance_trig, balance_flags_out] = fcn(state, target_volt_in, balance_flags_in, max_current_in, segments)
    % charge_ctrl 0 means charging, 1 means stop
    if state == 1 
        target_volt_out = target_volt_in;
        max_current_out = max_current_in;
        charge_ctrl = 0;
    else
        target_volt_out = 0;
        max_current_out = 0;
        charge_ctrl = 1;
    end
    
    if state == 2
        balance_trig = 1;
    else
        balance_trig = 0;
    end
    
    persistent balance_flags
    if isempty(balance_flags) %initialize persistant variable
        balance_flags = zeros(72, 1);
    end
    balance_flags_out = zeros(72, 1);
    
    if state == 8 % change state
        for i = 1:72
            balance_flags(i) = balance_flags_in(i);
        end
    end

    for i = 1:72
        balance_flags_out(i) = balance_flags(i);
    end

== matlab function accumulator/Charging/Charging Subsystem/MATLAB Function2 ==
  data: u input; H output; L output
function [H,L] = fcn(u)

    if u <= 255
        H = 0;
        L = u;
    else
        H = floor(u/256);
        L = mod(u, 256);

    end

end

== matlab function accumulator/Charging/Charging Subsystem/MATLAB Function3 ==
  data: u input; H output; L output
function [H,L] = fcn(u)

if u <= 255
    H = 0;
    L = u;

else
    H = floor(u/256);
    L = mod(u, 256);
    
end


end

== matlab function accumulator/Charging/Charging Subsystem/Balancing Subsystem/MATLAB Function ==
  data: balance_trig input; flags input; flags_1_out output; flags_2_out output; segments input
function [flags_1_out, flags_2_out] = fcn(balance_trig, flags, segments)
    flags_1 = zeros(64, 1, 'uint8');
    flags_2 = zeros(64, 1, 'uint8');

    if balance_trig == 1
        for segment = 0:3
            if segment < segments
                for cell = 1:12
                    flags_1(segment * 16 + cell) = flags(segment * 12 + cell);
                end
            end
        end
        for segment = 4:5
            if segment < segments
                for cell = 1:12
                    flags_2(segment * 16 + cell) = flags(segment * 12 + cell);
                end
            end
        end
    end
    
    flags_1_out = zeros(8, 1, 'uint8');
    flags_2_out = zeros(8, 1, 'uint8');
    for byte = 1:8
        for bit = 1:8
            flags_1_out(byte) = flags_1_out(byte) + flags_1((byte - 1) * 8 + bit) * 2^(8-bit);
            flags_2_out(byte) = flags_2_out(byte) + flags_2((byte - 1) * 8 + bit) * 2^(8-bit);
        end
    end
